simulink model "kontrol_nelin_svi"  (R2020a)
settings: Solver=ode4  StartTime=0.0  StopTime=tfin  FixedStep=1  RelTol=1e-3  EnableMultiTasking=on
values from neighbouring files (symbols this model uses):
  Ca = 1e-6    (= 1e-06)    [dec_stat_dek.m]    (also in dec_w0_dek.m; dec_zanemarivanje.m; hinf.m; inverzija_potpuna.m)
  Cb = 1e-6    (= 1e-06)    [dec_stat_dek.m]    (also in dec_w0_dek.m; dec_zanemarivanje.m; hinf.m; inverzija_potpuna.m)
  Fae = 1/60    (= 0.0166666666667)    [dec_stat_dek.m]    (also in dec_w0_dek.m; dec_zanemarivanje.m; hinf.m; inverzija_potpuna.m)
  Fastep = 0.01*Fae    (= 0.000166666666667)    [kontrola_nelin_svi_matlab.m]
  Fbe = 2/60    (= 0.0333333333333)    [dec_stat_dek.m]    (also in dec_w0_dek.m; dec_zanemarivanje.m; hinf.m; inverzija_potpuna.m)
  Fbstep = 0.01*Fbe    (= 0.000333333333333)    [kontrola_nelin_svi_matlab.m]
  kv = 0.01    [dec_stat_dek.m]    (also in dec_w0_dek.m; dec_zanemarivanje.m; hinf.m; inverzija_potpuna.m)
  kw = 1e-14    [dec_stat_dek.m]    (also in dec_w0_dek.m; dec_zanemarivanje.m; hinf.m; inverzija_potpuna.m)
  pHe = -log10(H_plus_e)    [dec_stat_dek.m]    (also in dec_w0_dek.m; dec_zanemarivanje.m; hinf.m; inverzija_potpuna.m)
  pHstep = 0.0596    [kontrola_nelin_dec_zan_matlab.m]    (also in kontrola_nelin_svi_matlab.m = 5.96e-05)
  tu1_step1 = 1000    [kontrola_nelin_dec_zan_matlab.m]    (also in kontrola_nelin_svi_matlab.m)
  tu1_step2 = 3000    [kontrola_nelin_dec_zan_matlab.m]    (also in kontrola_nelin_svi_matlab.m = 10000)
  tu2_step1 = 5000    [kontrola_nelin_dec_zan_matlab.m]    (also in kontrola_nelin_svi_matlab.m = 1000)
  tu2_step2 = 7000    [kontrola_nelin_dec_zan_matlab.m]    (also in kontrola_nelin_svi_matlab.m = 10000)
  V = 30    [dec_stat_dek.m]    (also in dec_w0_dek.m; dec_zanemarivanje.m; hinf.m; inverzija_potpuna.m)
  xa0 = xae    (= 3.33333333333e-07)    [kontrola_nelin_dec_zan_matlab.m]    (also in kontrola_nelin_svi_matlab.m)
  xae = Fae*Ca/(Fae+Fbe)    (= 3.33333333333e-07)    [dec_stat_dek.m]    (also in dec_w0_dek.m; dec_zanemarivanje.m; hinf.m; inverzija_potpuna.m)
  xastep = 2.0819e-08    [kontrola_nelin_dec_zan_matlab.m]    (also in kontrola_nelin_svi_matlab.m = 2.274336e-08)
  xb0 = xbe    (= 5.55555555556e-07)    [kontrola_nelin_dec_zan_matlab.m]    (also in kontrola_nelin_svi_matlab.m)
undefined symbols (not defined in the file or in its folder): magnitude
libraries: cstblocks x5
settings Model: Creator=Sanja  LastModifiedBy=cactoss
settings DataIOCC: LimitDataPoints=on  SaveFormat=Array  ReturnWorkspaceOutputs=off
settings OptimizationCC: LifeSpan=inf
settings DebuggingCC: UnderspecifiedInitializationDetection=Classic  MergeDetectMultiDrivingBlocksExec=none  SolverPrmCheckMsg=warning  SFUnexpectedBacktrackingDiag=warning  SFNoUnconditionalDefaultTransitionDiag=warning  SFExecutionAtInitializationDiag=none  ArithmeticOperatorsInVariantConditions=warning
settings HardwareCC: ProdBitPerPointer=32  ProdBitPerSizeT=32  ProdBitPerPtrDiffT=32  ProdLargestAtomicFloat=None  ProdIntDivRoundTo=Undefined  ProdEndianess=Unspecified  ProdWordSize=32  ProdHWDeviceType=32-bit Generic
settings ModelReferenceCC: PropagateSignalLabelsOutOfModel=off
settings SFSimCC: SimUseLocalCustomCode=off  CustomCodeUndefinedFunction=UseInterfaceOnly
settings RTWCC: RTWUseLocalCustomCode=off
settings CodeAppCC: StateflowObjectComments=on
settings GRTTargetCC: TargetLangStandard=C89/C90 (ANSI)
settings ConfigComp: CovMetricSettings=dw  CovHtmlReporting=on  CovSaveCumulativeToWorkspaceVar=on  CovSaveSingleToWorkspaceVar=on  CovExternalEMLEnable=off

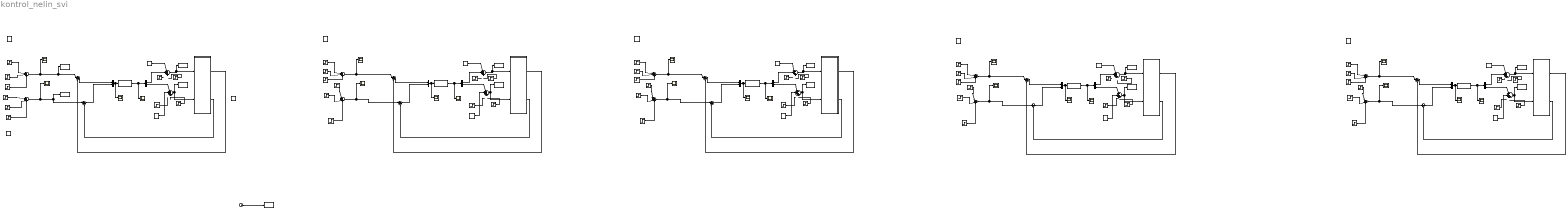
== system kontrol_nelin_svi ==
  note: Multivarijabilan Hinf Kontroler
  note: Decentralizovan kontroler, zanemarivanje sprežnih elemenata
  note: nelinearan sistem bi trebalo da se nalazi u nominalnom režimu.
  note: nelinearan sistem bi trebalo da se nalazi u nominalnom režimu.
  note: nelinearan sistem bi trebalo da se nalazi u nominalnom režimu.
  note: Decentralizovan kontroler, statičko dekuplovanje
  note: Decentralizovan kontroler, dekuplovanje na učestanosti propusnog opsega
  note: nelinearan sistem bi trebalo da se nalazi u nominalnom režimu.
  note: nelinearan sistem bi trebalo da se nalazi u nominalnom režimu.
  note: Decentralizovan kontroler, dekuplovanje sa potpunom inverzijom dinamike
  Clock : Clock
  Constant{,4,8,12,15} (5 alike) : Constant  Value=Fae
  Constant{1,5,9,13,16} (5 alike) : Constant  Value=Fbe
  Constant{2,6,10..11,14} (5 alike) : Constant  Value=pHe
  Constant3 : Constant  Value=xae
  Constant7 : Constant  Value=xae
  Demux{,1..4} (5 alike) : Demux  Outputs=2
  Kraj step pH{,1..4} (5 alike) : Step  Time=tu1_step2  After=-pHstep  SampleTime=0
  Kraj step xa{,1..4} (5 alike) : Step  Time=tu2_step2  After=-xastep  SampleTime=0
  LTI System1 : cstblocks/LTI System  sys=K_dec_z  IC=[]
  LTI System2 : cstblocks/LTI System  sys=K_dec_stat  IC=[]
  LTI System3 : cstblocks/LTI System  sys=K_dec_w0  IC=[]
  LTI System4 : cstblocks/LTI System  sys=K_hinf  IC=[]
  LTI System5 : cstblocks/LTI System  sys=K_inv  IC=[]
  Mux{,1..4} (5 alike) : Mux  Inputs=2
  Scope{,1..19} (20 alike) : Scope
  Step Fa{,1..4} (5 alike) : Step  Time=tu1_step1  After=Fastep  SampleTime=0
  Step Fa kraj{,1..4} (5 alike) : Step  Time=tu1_step2  After=-Fastep  SampleTime=0
  Step Fb{,1..4} (5 alike) : Step  Time=tu1_step1  After=Fbstep  SampleTime=0
  Step Fb kraj{,1..4} (5 alike) : Step  Time=tu1_step2  After=-Fbstep  SampleTime=0
  Step pH{,1..4} (5 alike) : Step  Time=tu1_step1  After=pHstep  SampleTime=0
  Step xa{,1..4} (5 alike) : Step  Time=tu2_step1  After=xastep  SampleTime=0
  Subsystem1 : Subsystem
  Subsystem2 : Subsystem
  Subsystem3 : Subsystem
  Subsystem4 : Subsystem
  Subsystem5 : Subsystem
  Sum{,1,6..7,12..13,18..19,24..25} (10 alike) : Sum  Inputs=|+++
  Sum{4..5,10..11,16..17,22..23,28..29} (10 alike) : Sum  Inputs=|++++
  Sum{2..3,8..9,14..15,20..21,26..27} (10 alike) : Sum  Inputs=|+-
  To Workspace : ToWorkspace  VariableName=Fa_dec_stat_out  SampleTime=-1
  To Workspace1 : ToWorkspace  VariableName=Fb_hinf_out  SampleTime=-1
  To Workspace10 : ToWorkspace  VariableName=Fb_inv_out  SampleTime=-1
  To Workspace11 : ToWorkspace  VariableName=Fb_dec_w0_out  SampleTime=-1
  To Workspace12 : ToWorkspace  VariableName=Fa_inv_out  SampleTime=-1
  To Workspace2 : ToWorkspace  VariableName=Fb_dec_stat_out  SampleTime=-1
  To Workspace3 : ToWorkspace  VariableName=Fa_hinf_out  SampleTime=-1
  To Workspace4 : ToWorkspace  VariableName=t_out  SampleTime=-1
  To Workspace5 : ToWorkspace  VariableName=Fa_dec_z_out  SampleTime=-1
  To Workspace6 : ToWorkspace  VariableName=pH_ref_out  SampleTime=-1
  To Workspace7 : ToWorkspace  VariableName=Fb_dec_z_out  SampleTime=-1
  To Workspace8 : ToWorkspace  VariableName=xa_ref_out  SampleTime=-1
  To Workspace9 : ToWorkspace  VariableName=Fa_dec_w0_out  SampleTime=-1
  pHe{,1..4} (5 alike) : Step  Time=0  After=pHe  SampleTime=0
  xae{,1..4} (5 alike) : Step  Time=0  After=xae  SampleTime=0
  wires:
  Clock/1 -> To Workspace4/1
  Demux/1 -> Sum4/2
  Sum3/1 -> Mux/2
  Sum2/1 -> Mux/1
  Sum/1 -> Scope2/1, Sum2/1
  Sum1/1 -> Scope3/1, Sum3/1
  Subsystem1/1(pH1) -> Sum2/2
  Subsystem1/2(xa) -> Sum3/2
  Mux/1 -> Scope1/1, LTI System2/1
  LTI System2/1 -> Scope/1, Demux/1
  Sum4/1 -> Subsystem1/1(Fa1), To Workspace/1
  Constant/1 -> Sum4/1
  Demux/2 -> Sum5/1
  Constant1/1 -> Sum5/2
  Sum5/1 -> To Workspace2/1, Subsystem1/2(Fb1)
  pHe/1 -> Sum/1
  xae/1 -> Sum1/1
  Step xa/1 -> Sum1/2
  Kraj step xa/1 -> Sum1/3
  Sum6/1 -> Scope6/1, To Workspace6/1, Sum8/1
  Kraj step xa1/1 -> Sum7/3
  Sum11/1 -> To Workspace7/1, Subsystem2/2(Fb1)
  Step xa1/1 -> Sum7/2
  pHe1/1 -> Sum6/1
  Subsystem2/1(pH1) -> Sum8/2
  Constant4/1 -> Sum10/1
  Sum7/1 -> Scope7/1, To Workspace8/1, Sum9/1
  Sum9/1 -> Mux1/2
  Sum8/1 -> Mux1/1
  Sum10/1 -> Subsystem2/1(Fa1), To Workspace5/1
  Demux1/1 -> Sum10/2
  Subsystem2/2(xa) -> Sum9/2
  xae1/1 -> Sum7/1
  Demux1/2 -> Sum11/1
  Mux1/1 -> Scope5/1, LTI System1/1
  Constant5/1 -> Sum11/2
  LTI System1/1 -> Scope4/1, Demux1/1
  Sum12/1 -> Scope10/1, Sum14/1
  Kraj step xa2/1 -> Sum13/3
  Sum17/1 -> To Workspace11/1, Subsystem3/2(Fb1)
  Step xa2/1 -> Sum13/2
  pHe2/1 -> Sum12/1
  Subsystem3/1(pH1) -> Sum14/2
  Constant8/1 -> Sum16/1
  Sum13/1 -> Scope11/1, Sum15/1
  Sum15/1 -> Mux2/2
  Sum14/1 -> Mux2/1
  Sum16/1 -> Subsystem3/1(Fa1), To Workspace9/1
  Subsystem3/2(xa) -> Sum15/2
  Constant9/1 -> Sum17/2
  LTI System3/1 -> Scope8/1, Demux2/1
  xae2/1 -> Sum13/1
  Demux2/2 -> Sum17/1
  Mux2/1 -> Scope9/1, LTI System3/1
  Demux2/1 -> Sum16/2
  LTI System4/1 -> Scope14/1, Demux3/1
  Constant13/1 -> Sum23/2
  Demux3/1 -> Sum22/2
  Demux3/2 -> Sum23/1
  xae3/1 -> Sum19/1
  Sum19/1 -> Scope13/1, Sum21/1
  pHe3/1 -> Sum18/1
  Step xa3/1 -> Sum19/2
  Subsystem4/2(xa) -> Sum21/2
  Sum20/1 -> Mux3/1
  Sum22/1 -> Subsystem4/1(Fa1), To Workspace3/1
  Constant12/1 -> Sum22/1
  Subsystem4/1(pH1) -> Sum20/2
  Sum23/1 -> To Workspace1/1, Subsystem4/2(Fb1)
  Sum21/1 -> Mux3/2
  Sum18/1 -> Scope12/1, Sum20/1
  Mux3/1 -> Scope15/1, LTI System4/1
  Kraj step xa3/1 -> Sum19/3
  Kraj step xa4/1 -> Sum25/3
  Mux4/1 -> Scope19/1, LTI System5/1
  Sum27/1 -> Mux4/2
  Sum29/1 -> To Workspace10/1, Subsystem5/2(Fb1)
  Subsystem5/1(pH1) -> Sum26/2
  Constant15/1 -> Sum28/1
  Sum26/1 -> Mux4/1
  Sum28/1 -> Subsystem5/1(Fa1), To Workspace12/1
  Subsystem5/2(xa) -> Sum27/2
  Step xa4/1 -> Sum25/2
  Sum25/1 -> Scope17/1, Sum27/1
  pHe4/1 -> Sum24/1
  Demux4/2 -> Sum29/1
  LTI System5/1 -> Scope18/1, Demux4/1
  Sum24/1 -> Scope16/1, Sum26/1
  Constant16/1 -> Sum29/2
  Demux4/1 -> Sum28/2
  xae4/1 -> Sum25/1
  Step pH4/1 -> Sum24/2
  Kraj step pH4/1 -> Sum24/3
  Step pH1/1 -> Sum6/2
  Kraj step pH1/1 -> Sum6/3
  Step pH/1 -> Sum/2
  Kraj step pH/1 -> Sum/3
  Step pH2/1 -> Sum12/2
  Kraj step pH2/1 -> Sum12/3
  Step pH3/1 -> Sum18/2
  Kraj step pH3/1 -> Sum18/3
  Step Fa/1 -> ?
  Step Fa kraj/1 -> ?
  Step Fb/1 -> ?
  Step Fb kraj/1 -> ?
  Step Fa1/1 -> ?
  Step Fa kraj1/1 -> ?
  Step Fa2/1 -> ?
  Step Fa kraj2/1 -> ?
  Step Fa3/1 -> ?
  Step Fa kraj3/1 -> ?
  Step Fb3/1 -> ?
  Step Fb kraj3/1 -> ?
  Step Fa4/1 -> ?
  Step Fa kraj4/1 -> ?
  Step Fb1/1 -> ?
  Step Fb kraj1/1 -> ?
  Step Fb2/1 -> ?
  Step Fb kraj2/1 -> ?
  Step Fb4/1 -> ?
  Step Fb kraj4/1 -> ?

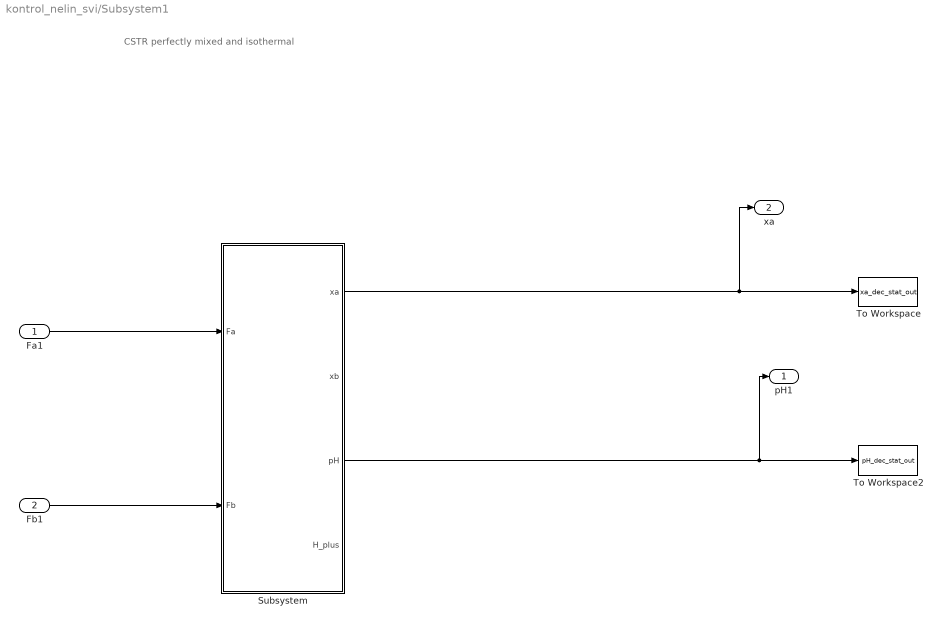
== system kontrol_nelin_svi/Subsystem1 ==
  note: CSTR perfectly mixed and isothermal
  Fa1 : Inport
  Fb1 : Inport  Port=2
  Subsystem : Subsystem
  To Workspace : ToWorkspace  VariableName=xa_dec_stat_out  SampleTime=-1
  To Workspace2 : ToWorkspace  VariableName=pH_dec_stat_out  SampleTime=-1
  pH1 : Outport
  xa : Outport  Port=2
  wires:
  Subsystem/3(pH) -> pH1/1, To Workspace2/1
  Subsystem/1(xa) -> xa/1, To Workspace/1
  Fb1/1 -> Subsystem/2(Fb)
  Fa1/1 -> Subsystem/1(Fa)

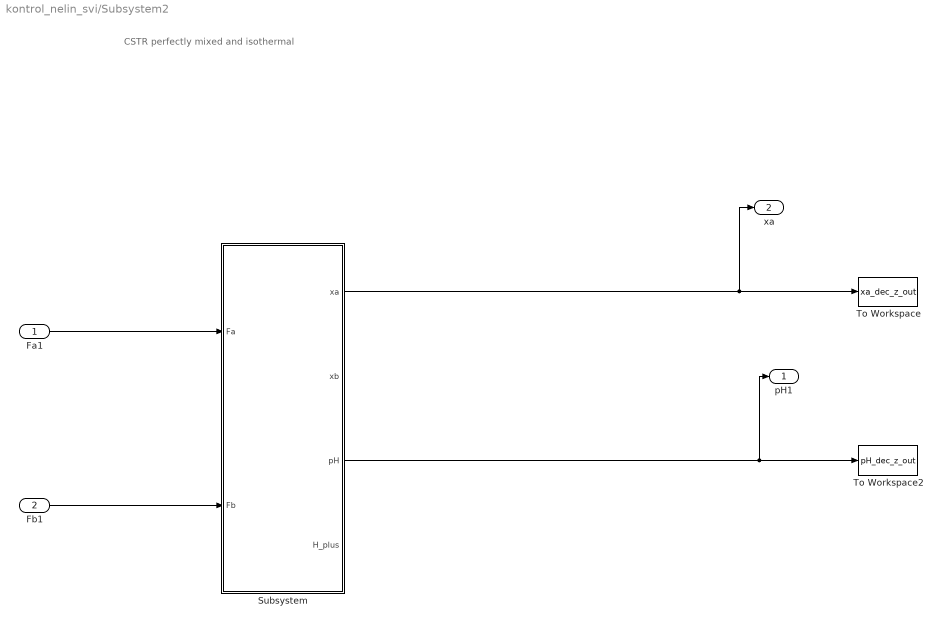
== system kontrol_nelin_svi/Subsystem2 ==
  note: CSTR perfectly mixed and isothermal
  Fa1 : Inport
  Fb1 : Inport  Port=2
  Subsystem : Subsystem
  To Workspace : ToWorkspace  VariableName=xa_dec_z_out  SampleTime=-1
  To Workspace2 : ToWorkspace  VariableName=pH_dec_z_out  SampleTime=-1
  pH1 : Outport
  xa : Outport  Port=2
  wires:
  Subsystem/3(pH) -> pH1/1, To Workspace2/1
  Subsystem/1(xa) -> xa/1, To Workspace/1
  Fb1/1 -> Subsystem/2(Fb)
  Fa1/1 -> Subsystem/1(Fa)

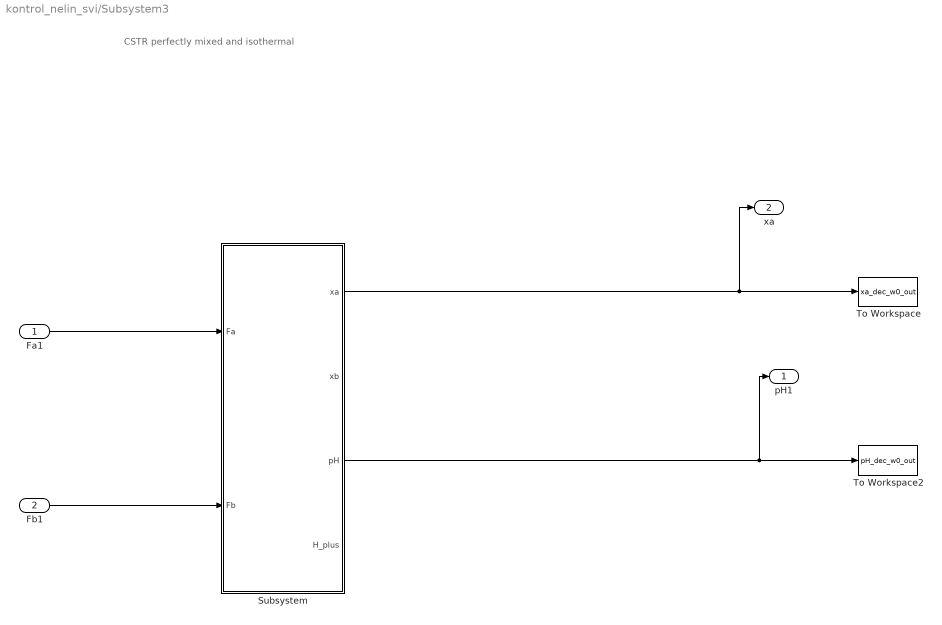
== system kontrol_nelin_svi/Subsystem3 ==
  note: CSTR perfectly mixed and isothermal
  Fa1 : Inport
  Fb1 : Inport  Port=2
  Subsystem : Subsystem
  To Workspace : ToWorkspace  VariableName=xa_dec_w0_out  SampleTime=-1
  To Workspace2 : ToWorkspace  VariableName=pH_dec_w0_out  SampleTime=-1
  pH1 : Outport
  xa : Outport  Port=2
  wires:
  Subsystem/3(pH) -> pH1/1, To Workspace2/1
  Subsystem/1(xa) -> xa/1, To Workspace/1
  Fb1/1 -> Subsystem/2(Fb)
  Fa1/1 -> Subsystem/1(Fa)

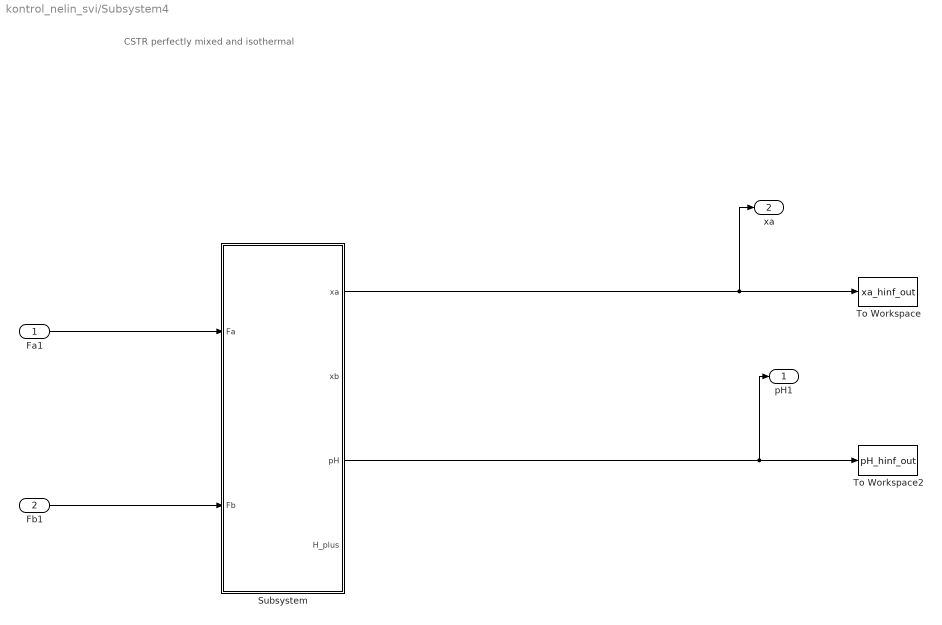
== system kontrol_nelin_svi/Subsystem4 ==
  note: CSTR perfectly mixed and isothermal
  Fa1 : Inport
  Fb1 : Inport  Port=2
  Subsystem : Subsystem
  To Workspace : ToWorkspace  VariableName=xa_hinf_out  SampleTime=-1
  To Workspace2 : ToWorkspace  VariableName=pH_hinf_out  SampleTime=-1
  pH1 : Outport
  xa : Outport  Port=2
  wires:
  Subsystem/3(pH) -> pH1/1, To Workspace2/1
  Subsystem/1(xa) -> xa/1, To Workspace/1
  Fb1/1 -> Subsystem/2(Fb)
  Fa1/1 -> Subsystem/1(Fa)

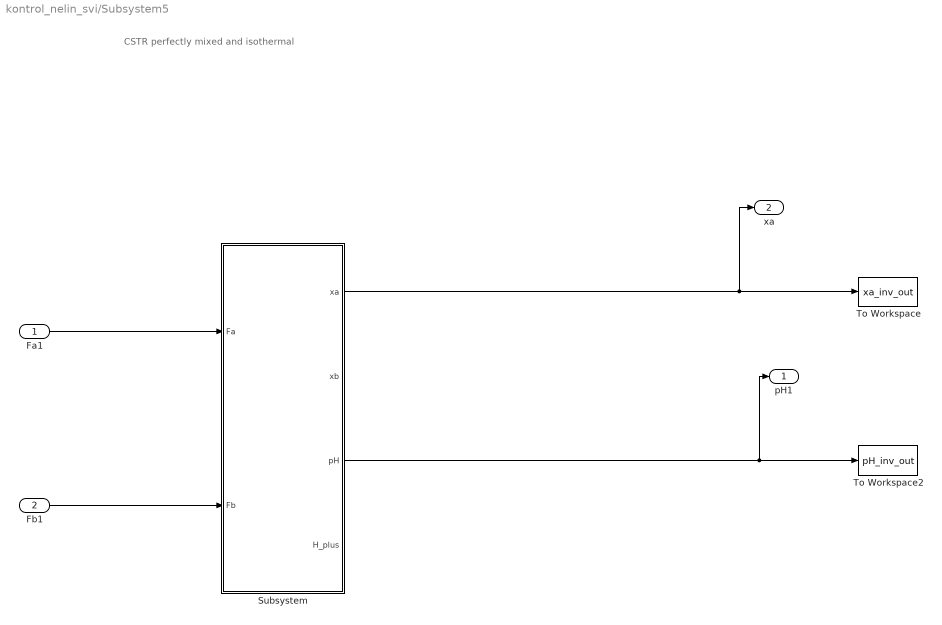
== system kontrol_nelin_svi/Subsystem5 ==
  note: CSTR perfectly mixed and isothermal
  Fa1 : Inport
  Fb1 : Inport  Port=2
  Subsystem : Subsystem
  To Workspace : ToWorkspace  VariableName=xa_inv_out  SampleTime=-1
  To Workspace2 : ToWorkspace  VariableName=pH_inv_out  SampleTime=-1
  pH1 : Outport
  xa : Outport  Port=2
  wires:
  Subsystem/3(pH) -> pH1/1, To Workspace2/1
  Subsystem/1(xa) -> xa/1, To Workspace/1
  Fb1/1 -> Subsystem/2(Fb)
  Fa1/1 -> Subsystem/1(Fa)

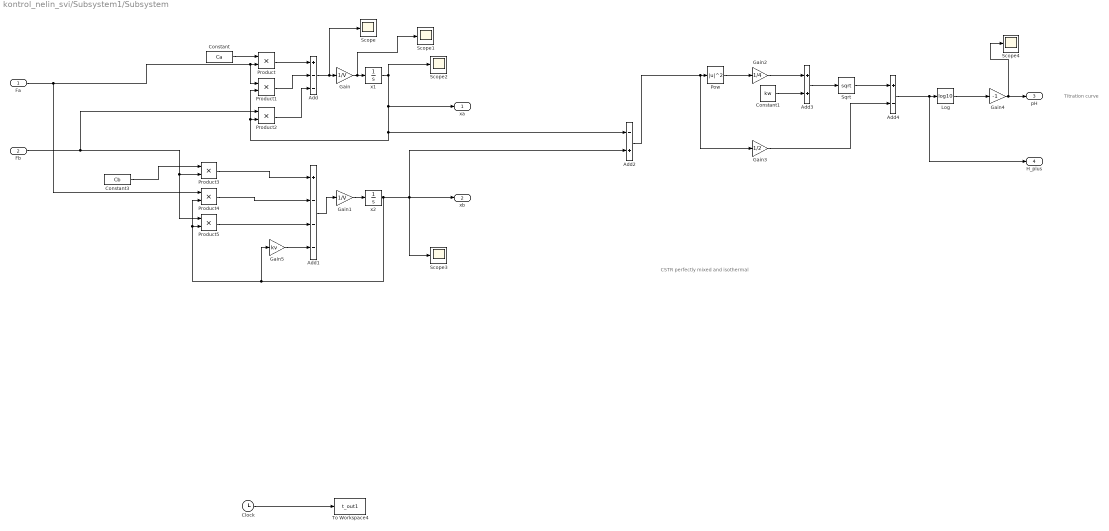
== system kontrol_nelin_svi/Subsystem1/Subsystem ==
  note: Titration curve
  note: CSTR perfectly mixed and isothermal
  Fa : Inport
  Fb : Inport  Port=2
  Add : Sum  Inputs=+--
  Add1 : Sum  Inputs=+---
  Add2 : Sum  Inputs=-+
  Add3 : Sum
  Add4 : Sum  Inputs=+-
  Clock : Clock
  Constant : Constant  Value=Ca
  Constant1 : Constant  Value=kw
  Constant3 : Constant  Value=Cb
  Gain : Gain  Gain=1/V
  Gain1 : Gain  Gain=1/V
  Gain2 : Gain  Gain=1/4
  Gain3 : Gain  Gain=1/2
  Gain4 : Gain  Gain=-1
  Gain5 : Gain  Gain=kv
  Log : Math  Operator=log10  SaturateOnIntegerOverflow=on
  Pow : Math  Operator=magnitude^2  SignedPower=on  RndMeth=Zero  SaturateOnIntegerOverflow=on
  Product{,1..5} (6 alike) : Product
  Scope{,1..4} (5 alike) : Scope
  Sqrt : Sqrt  SaturateOnIntegerOverflow=on
  To Workspace4 : ToWorkspace  VariableName=t_out1  SampleTime=-1
  x1 : Integrator  InitialCondition=xa0
  x2 : Integrator  InitialCondition=xb0
  xa : Outport
  xb : Outport  Port=2
  pH : Outport  Port=3
  H_plus : Outport  Port=4
  wires:
  Fb/1 -> Product5/1, Product3/2, Product2/1
  Constant3/1 -> Product3/1
  Product3/1 -> Add1/1
  Product5/1 -> Add1/3
  Product4/1 -> Add1/2
  x1/1 -> Scope2/1, Product1/2, Product2/2, Add2/1, xa/1
  Product2/1 -> Add/3
  x2/1 -> Add2/2, xb/1, Scope3/1, Gain5/1, Product4/2, Product5/2
  Add1/1 -> Gain1/1
  Gain1/1 -> x2/1
  Gain/1 -> Scope1/1, x1/1
  Fa/1 -> Product1/1, Product/2, Product4/1
  Product1/1 -> Add/2
  Product/1 -> Add/1
  Add/1 -> Scope/1, Gain/1
  Constant/1 -> Product/1
  Add2/1 -> Gain3/1, Pow/1
  Pow/1 -> Gain2/1
  Gain2/1 -> Add3/1
  Constant1/1 -> Add3/2
  Add3/1 -> Sqrt/1
  Sqrt/1 -> Add4/1
  Gain3/1 -> Add4/2
  Add4/1 -> H_plus/1, Log/1
  Log/1 -> Gain4/1
  Gain4/1 -> Scope4/1, pH/1
  Clock/1 -> To Workspace4/1
  Gain5/1 -> Add1/4

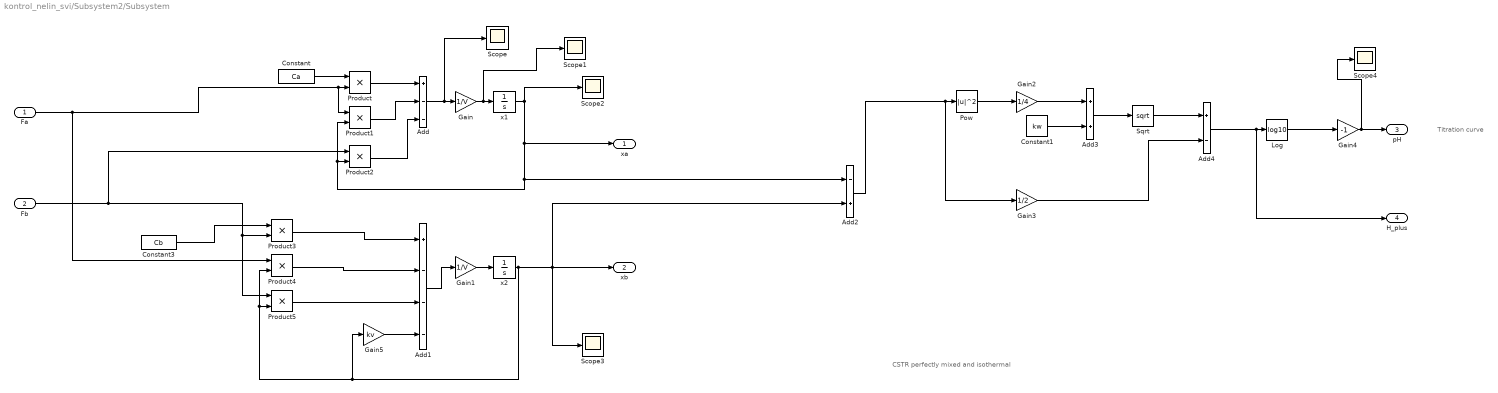
== system kontrol_nelin_svi/Subsystem2/Subsystem ==
  note: Titration curve
  note: CSTR perfectly mixed and isothermal
  Fa : Inport
  Fb : Inport  Port=2
  Add : Sum  Inputs=+--
  Add1 : Sum  Inputs=+---
  Add2 : Sum  Inputs=-+
  Add3 : Sum
  Add4 : Sum  Inputs=+-
  Constant : Constant  Value=Ca
  Constant1 : Constant  Value=kw
  Constant3 : Constant  Value=Cb
  Gain : Gain  Gain=1/V
  Gain1 : Gain  Gain=1/V
  Gain2 : Gain  Gain=1/4
  Gain3 : Gain  Gain=1/2
  Gain4 : Gain  Gain=-1
  Gain5 : Gain  Gain=kv
  Log : Math  Operator=log10  SaturateOnIntegerOverflow=on
  Pow : Math  Operator=magnitude^2  SignedPower=on  RndMeth=Zero  SaturateOnIntegerOverflow=on
  Product{,1..5} (6 alike) : Product
  Scope{,1..4} (5 alike) : Scope
  Sqrt : Sqrt  SaturateOnIntegerOverflow=on
  x1 : Integrator  InitialCondition=xa0
  x2 : Integrator  InitialCondition=xb0
  xa : Outport
  xb : Outport  Port=2
  pH : Outport  Port=3
  H_plus : Outport  Port=4
  wires:
  Fb/1 -> Product5/1, Product3/2, Product2/1
  Constant3/1 -> Product3/1
  Product3/1 -> Add1/1
  Product5/1 -> Add1/3
  Product4/1 -> Add1/2
  x1/1 -> Scope2/1, Product1/2, Product2/2, Add2/1, xa/1
  Product2/1 -> Add/3
  x2/1 -> Add2/2, xb/1, Scope3/1, Gain5/1, Product4/2, Product5/2
  Add1/1 -> Gain1/1
  Gain1/1 -> x2/1
  Gain/1 -> Scope1/1, x1/1
  Fa/1 -> Product1/1, Product/2, Product4/1
  Product1/1 -> Add/2
  Product/1 -> Add/1
  Add/1 -> Scope/1, Gain/1
  Constant/1 -> Product/1
  Add2/1 -> Gain3/1, Pow/1
  Pow/1 -> Gain2/1
  Gain2/1 -> Add3/1
  Constant1/1 -> Add3/2
  Add3/1 -> Sqrt/1
  Sqrt/1 -> Add4/1
  Gain3/1 -> Add4/2
  Add4/1 -> H_plus/1, Log/1
  Log/1 -> Gain4/1
  Gain4/1 -> Scope4/1, pH/1
  Gain5/1 -> Add1/4

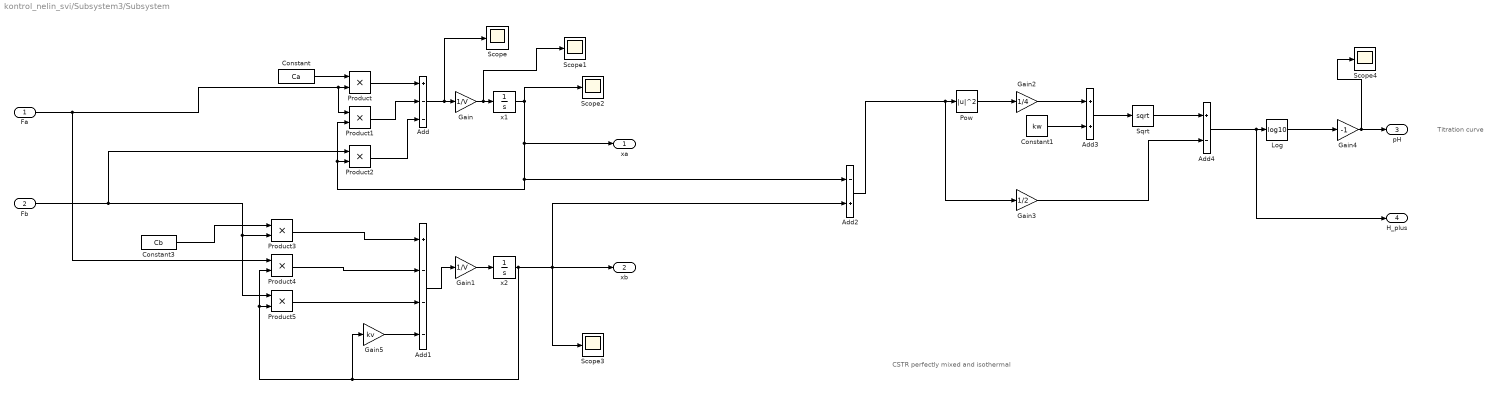
== system kontrol_nelin_svi/Subsystem3/Subsystem ==
  note: Titration curve
  note: CSTR perfectly mixed and isothermal
  Fa : Inport
  Fb : Inport  Port=2
  Add : Sum  Inputs=+--
  Add1 : Sum  Inputs=+---
  Add2 : Sum  Inputs=-+
  Add3 : Sum
  Add4 : Sum  Inputs=+-
  Constant : Constant  Value=Ca
  Constant1 : Constant  Value=kw
  Constant3 : Constant  Value=Cb
  Gain : Gain  Gain=1/V
  Gain1 : Gain  Gain=1/V
  Gain2 : Gain  Gain=1/4
  Gain3 : Gain  Gain=1/2
  Gain4 : Gain  Gain=-1
  Gain5 : Gain  Gain=kv
  Log : Math  Operator=log10  SaturateOnIntegerOverflow=on
  Pow : Math  Operator=magnitude^2  SignedPower=on  RndMeth=Zero  SaturateOnIntegerOverflow=on
  Product{,1..5} (6 alike) : Product
  Scope{,1..4} (5 alike) : Scope
  Sqrt : Sqrt  SaturateOnIntegerOverflow=on
  x1 : Integrator  InitialCondition=xa0
  x2 : Integrator  InitialCondition=xb0
  xa : Outport
  xb : Outport  Port=2
  pH : Outport  Port=3
  H_plus : Outport  Port=4
  wires:
  Fb/1 -> Product5/1, Product3/2, Product2/1
  Constant3/1 -> Product3/1
  Product3/1 -> Add1/1
  Product5/1 -> Add1/3
  Product4/1 -> Add1/2
  x1/1 -> Scope2/1, Product1/2, Product2/2, Add2/1, xa/1
  Product2/1 -> Add/3
  x2/1 -> Add2/2, xb/1, Scope3/1, Gain5/1, Product4/2, Product5/2
  Add1/1 -> Gain1/1
  Gain1/1 -> x2/1
  Gain/1 -> Scope1/1, x1/1
  Fa/1 -> Product1/1, Product/2, Product4/1
  Product1/1 -> Add/2
  Product/1 -> Add/1
  Add/1 -> Scope/1, Gain/1
  Constant/1 -> Product/1
  Add2/1 -> Gain3/1, Pow/1
  Pow/1 -> Gain2/1
  Gain2/1 -> Add3/1
  Constant1/1 -> Add3/2
  Add3/1 -> Sqrt/1
  Sqrt/1 -> Add4/1
  Gain3/1 -> Add4/2
  Add4/1 -> H_plus/1, Log/1
  Log/1 -> Gain4/1
  Gain4/1 -> Scope4/1, pH/1
  Gain5/1 -> Add1/4

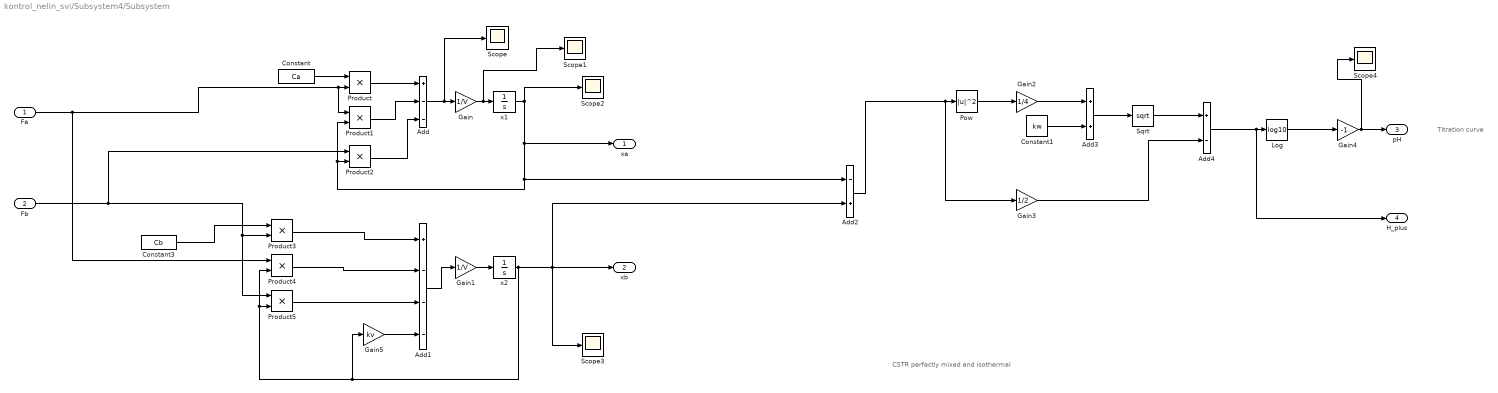
== system kontrol_nelin_svi/Subsystem4/Subsystem ==
  note: Titration curve
  note: CSTR perfectly mixed and isothermal
  Fa : Inport
  Fb : Inport  Port=2
  Add : Sum  Inputs=+--
  Add1 : Sum  Inputs=+---
  Add2 : Sum  Inputs=-+
  Add3 : Sum
  Add4 : Sum  Inputs=+-
  Constant : Constant  Value=Ca
  Constant1 : Constant  Value=kw
  Constant3 : Constant  Value=Cb
  Gain : Gain  Gain=1/V
  Gain1 : Gain  Gain=1/V
  Gain2 : Gain  Gain=1/4
  Gain3 : Gain  Gain=1/2
  Gain4 : Gain  Gain=-1
  Gain5 : Gain  Gain=kv
  Log : Math  Operator=log10  SaturateOnIntegerOverflow=on
  Pow : Math  Operator=magnitude^2  SignedPower=on  RndMeth=Zero  SaturateOnIntegerOverflow=on
  Product{,1..5} (6 alike) : Product
  Scope{,1..4} (5 alike) : Scope
  Sqrt : Sqrt  SaturateOnIntegerOverflow=on
  x1 : Integrator  InitialCondition=xa0
  x2 : Integrator  InitialCondition=xb0
  xa : Outport
  xb : Outport  Port=2
  pH : Outport  Port=3
  H_plus : Outport  Port=4
  wires:
  Fb/1 -> Product5/1, Product3/2, Product2/1
  Constant3/1 -> Product3/1
  Product3/1 -> Add1/1
  Product5/1 -> Add1/3
  Product4/1 -> Add1/2
  x1/1 -> Scope2/1, Product1/2, Product2/2, Add2/1, xa/1
  Product2/1 -> Add/3
  x2/1 -> Add2/2, xb/1, Scope3/1, Gain5/1, Product4/2, Product5/2
  Add1/1 -> Gain1/1
  Gain1/1 -> x2/1
  Gain/1 -> Scope1/1, x1/1
  Fa/1 -> Product1/1, Product/2, Product4/1
  Product1/1 -> Add/2
  Product/1 -> Add/1
  Add/1 -> Scope/1, Gain/1
  Constant/1 -> Product/1
  Add2/1 -> Gain3/1, Pow/1
  Pow/1 -> Gain2/1
  Gain2/1 -> Add3/1
  Constant1/1 -> Add3/2
  Add3/1 -> Sqrt/1
  Sqrt/1 -> Add4/1
  Gain3/1 -> Add4/2
  Add4/1 -> H_plus/1, Log/1
  Log/1 -> Gain4/1
  Gain4/1 -> Scope4/1, pH/1
  Gain5/1 -> Add1/4

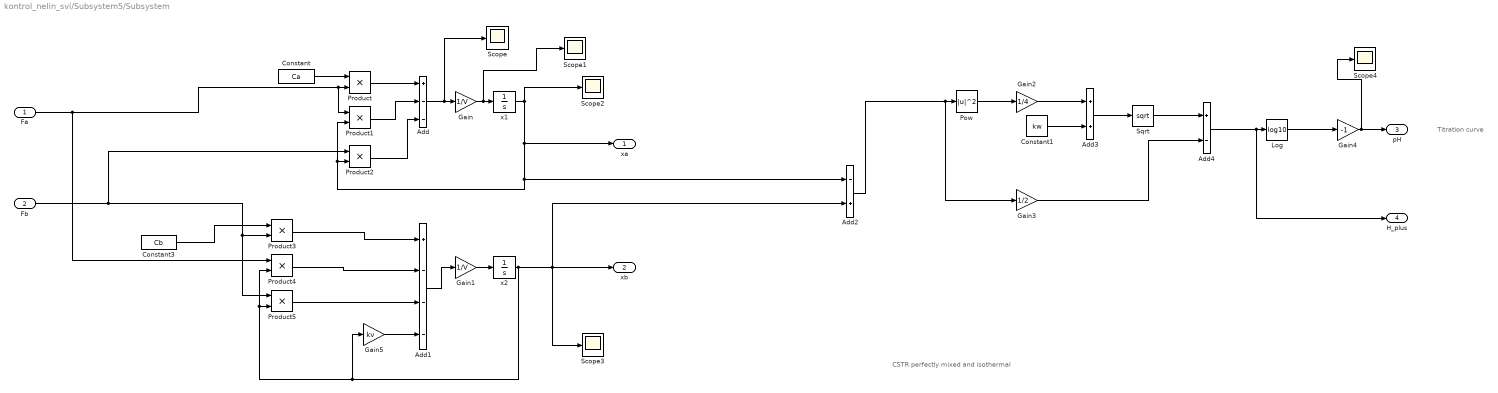
== system kontrol_nelin_svi/Subsystem5/Subsystem ==
  note: Titration curve
  note: CSTR perfectly mixed and isothermal
  Fa : Inport
  Fb : Inport  Port=2
  Add : Sum  Inputs=+--
  Add1 : Sum  Inputs=+---
  Add2 : Sum  Inputs=-+
  Add3 : Sum
  Add4 : Sum  Inputs=+-
  Constant : Constant  Value=Ca
  Constant1 : Constant  Value=kw
  Constant3 : Constant  Value=Cb
  Gain : Gain  Gain=1/V
  Gain1 : Gain  Gain=1/V
  Gain2 : Gain  Gain=1/4
  Gain3 : Gain  Gain=1/2
  Gain4 : Gain  Gain=-1
  Gain5 : Gain  Gain=kv
  Log : Math  Operator=log10  SaturateOnIntegerOverflow=on
  Pow : Math  Operator=magnitude^2  SignedPower=on  RndMeth=Zero  SaturateOnIntegerOverflow=on
  Product{,1..5} (6 alike) : Product
  Scope{,1..4} (5 alike) : Scope
  Sqrt : Sqrt  SaturateOnIntegerOverflow=on
  x1 : Integrator  InitialCondition=xa0
  x2 : Integrator  InitialCondition=xb0
  xa : Outport
  xb : Outport  Port=2
  pH : Outport  Port=3
  H_plus : Outport  Port=4
  wires:
  Fb/1 -> Product5/1, Product3/2, Product2/1
  Constant3/1 -> Product3/1
  Product3/1 -> Add1/1
  Product5/1 -> Add1/3
  Product4/1 -> Add1/2
  x1/1 -> Scope2/1, Product1/2, Product2/2, Add2/1, xa/1
  Product2/1 -> Add/3
  x2/1 -> Add2/2, xb/1, Scope3/1, Gain5/1, Product4/2, Product5/2
  Add1/1 -> Gain1/1
  Gain1/1 -> x2/1
  Gain/1 -> Scope1/1, x1/1
  Fa/1 -> Product1/1, Product/2, Product4/1
  Product1/1 -> Add/2
  Product/1 -> Add/1
  Add/1 -> Scope/1, Gain/1
  Constant/1 -> Product/1
  Add2/1 -> Gain3/1, Pow/1
  Pow/1 -> Gain2/1
  Gain2/1 -> Add3/1
  Constant1/1 -> Add3/2
  Add3/1 -> Sqrt/1
  Sqrt/1 -> Add4/1
  Gain3/1 -> Add4/2
  Add4/1 -> H_plus/1, Log/1
  Log/1 -> Gain4/1
  Gain4/1 -> Scope4/1, pH/1
  Gain5/1 -> Add1/4
